simulink model "A4T2"  (R2017a)
settings: Solver=VariableStepAuto  StartTime=0.0  StopTime=w_base  MaxStep=1e-4*w_base  RelTol=1e-3
values from neighbouring files (symbols this model uses):
  alpha_l = 4    [parameters.m]
  epsilon = (Lsigma+LM)/Lsigma    (= 6.36273701566)    [parameters.m]
  I_base = 1    [parameters.m]
  K = sqrt(3/2)    [parameters.m]
  ki = alpha_c*(R+Ra)    (= 11.8344493889)    [parameters.m]
  ki_speed = alpha_speed*alpha_speed*J    (= 0.9756347394)    [parameters.m]
  kp = alpha_c*Lsigma    (= 1.69441359229)    [parameters.m]
  kp_speed = alpha_speed*J    (= 6.98439238374)    [parameters.m]
  lambda = 1.5    [parameters.m]
  lambda_delta = 0.2*1    (= 0.2)    [parameters.m]
  Lsigma = 0.2426    [parameters.m]
  Ra = alpha_c*Lsigma-R    (= 1.58785359229)    [parameters.m]
  Ra_speed = alpha_speed*J-b    (= 6.48439238374)    [parameters.m]
  RR = 0.06151    [parameters.m]
  Rs = 0.04505    [parameters.m]
  V_base = 1    [parameters.m]
  w_base = 314.59    [parameters.m]
libraries: simulink x1
settings Model: Creator=Oskar  LastModifiedBy=Callum

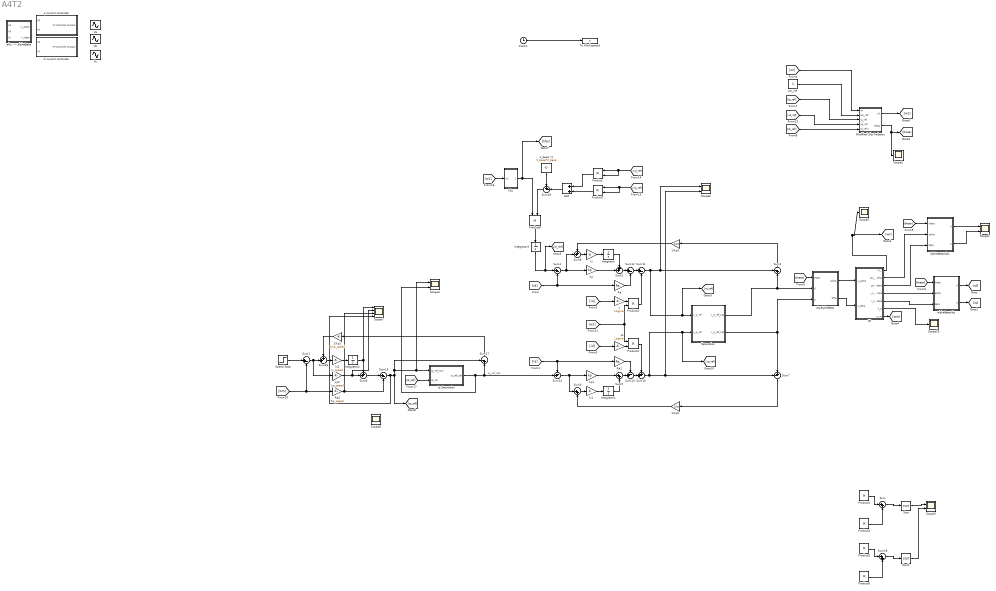
== system A4T2 ==
  note: iq_ref_sat
  1/kp1 : Gain  Gain=1/kp_speed
  1/kp2 : Gain  Gain=1/kp
  1/kp3 : Gain  Gain=1/kp
  Add : Sum
  Clock1 : Clock
  IM : Subsystem  mask{RR=0.06151, RS=0.04505, LM=1.301, Ls=0.2426, J=50, p=2, b_w1=0.5, b_w2=0}
      mask prompts: RR "Rr [p.u]"; RS "Rs [p.u]"; LM "Lm [p.u]"; Ls "Ls [p.u]"; J "J [p.u]"
  Integrator : Integrator
  Integrator1 : Integrator
  Integrator2 : Integrator
  Integrator3 : Integrator  InitialCondition=0.76863950807071483474250576479631  LimitOutput=on  UpperSaturationLimit=0.76863950807071483474250576479631  LowerSaturationLimit=0.1*I_base
  L : Gain  Gain=Lsigma
  L1 : Gain  Gain=Lsigma
  Modified Slip Relation : Subsystem
  Product{,1..8} (9 alike) : Product
  Ra : Gain  Gain=Ra
  Ra1 : Gain  Gain=Ra
  Ra2 : Gain  Gain=Ra_speed
  Saturation : Subsystem
  Scope{1,3..4,6,8} (5 alike) : Scope  NumInputPorts=2
  Scope10 : Scope
  Scope2 : Scope
  Scope5 : Scope
  Scope7 : Scope  NumInputPorts=4
  Speed Step : Step  Time=150  After=0.65  SampleTime=0
  Sqrt : Sqrt  SaturateOnIntegerOverflow=on
  Sqrt1 : Sqrt  SaturateOnIntegerOverflow=on
  Sum{,5,9,18} (4 alike) : Sum  Inputs=|++
  Sum{1,4,11..12,15} (5 alike) : Sum  Inputs=|+-
  Sum{3,6,8,10,16} (5 alike) : Sum  Inputs=++|
  Sum{2,7,13..14,17} (5 alike) : Sum  Inputs=-+|
  Sum19 : Sum  Inputs=+-|
  To Workspace1 : ToWorkspace  VariableName=t
      settings: MaxDataPoints=100000
  V_base^2 : Constant  Value=V_base*V_base
  Va : Sin  SampleTime=0
  Vb : Sin  Phase=2*pi/3  SampleTime=0
  Vc : Sin  Phase=4*pi/3  SampleTime=0
  abc --> alphaBeta : Subsystem
  alphaBeta/dq : Subsystem
  alphaBeta/dq1 : Subsystem
  d current controller : Subsystem
  dq/alphaBeta : Subsystem
  iq Saturation : Subsystem
  kfw : Subsystem
  ki : Gain  Gain=ki
  ki1 : Gain  Gain=ki
  ki2 : Gain  Gain=ki_speed
  kp : Gain  Gain=kp
  kp1 : Gain  Gain=kp
  kp2 : Gain  Gain=kp_speed
  psi_ref : Constant
  q current controller : Subsystem
  wires:
  Clock1/1 -> To Workspace1/1
  dq/alphaBeta/1(alpha) -> IM/1(u_alpha)
  dq/alphaBeta/2(beta) -> IM/2(u_beta)
  IM/4(i_s_s_alpha) -> alphaBeta/dq/2(alpha)
  IM/5(i_s_s_beta) -> alphaBeta/dq/3("beta ")
  alphaBeta/dq/1(d) -> [id]
  ki/1 -> Integrator/1
  Sum4/1 -> kp/1, Sum8/2
  [id] -> Ra/1, Sum4/2
  Sum14/1 -> kp1/1, Sum9/1
  ki1/1 -> Integrator1/1
  kp1/1 -> Sum5/1
  Integrator1/1 -> Sum5/2
  Sum7/1 -> 1/kp2/1
  Sum2/1 -> 1/kp3/1
  kp/1 -> Sum3/2
  Integrator/1 -> Sum3/1
  Sum8/1 -> ki/1
  1/kp3/1 -> Sum8/1
  Sum9/1 -> ki1/1
  1/kp2/1 -> Sum9/2
  [iq] -> L/1
  [id] -> L1/1
  Sum3/1 -> Sum12/1
  Sum12/1 -> Sum11/1
  Ra/1 -> Sum12/2
  Sum5/1 -> Sum13/2
  Sum13/1 -> Sum10/2
  Ra1/1 -> Sum13/1
  [iq] -> Ra1/1, Sum14/1
  IM/1(w_r) -> Scope5/1, [wr]
  Modified Slip Relation/2(theta) -> Scope2/1, [theta]
  [theta] -> dq/alphaBeta/1(theta)
  [theta] -> alphaBeta/dq/1(theta)
  Sum15/1 -> Scope7/4, Scope4/1, iq Saturation/1(iq_ref_nom), Sum17/1, [iq_ref]
  L/1 -> Product3/1
  Product3/1 -> Sum11/2
  [w1] -> Product3/2, Product4/1
  L1/1 -> Product4/2
  Product4/1 -> Sum10/1
  Saturation/1(v_d_ref_sat) -> Sum2/2, dq/alphaBeta/2(d)
  Saturation/2(v_q_ref_sat) -> dq/alphaBeta/3("q "), Sum7/2
  IM/2(psi_r_alpha) -> alphaBeta/dq1/2(alpha)
  IM/3(psi_r_beta) -> alphaBeta/dq1/3("beta ")
  [theta] -> alphaBeta/dq1/1(theta)
  Modified Slip Relation/1(w1) -> [w1]
  Speed Step/1 -> Sum1/1
  IM/7(w_m) -> [wm]
  [wm] -> Sum1/2, Ra2/1
  ki2/1 -> Integrator2/1
  Sum16/1 -> ki2/1
  kp2/1 -> Scope7/2, Sum6/2
  Integrator2/1 -> Sum6/1, Scope7/1
  Sum1/1 -> kp2/1, Sum16/2
  Sum6/1 -> Sum15/1
  Ra2/1 -> Sum15/2, Scope7/3
  1/kp1/1 -> Sum16/1
  Sum17/1 -> 1/kp1/1
  IM/6(T_e) -> Scope10/1
  Sum/1 -> Sqrt/1
  Product1/1 -> Sum/1
  Product2/1 -> Sum/2
  Sqrt/1 -> Scope3/1
  Sum18/1 -> Sqrt1/1
  Product6/1 -> Sum18/2
  Product5/1 -> Sum18/1
  Sqrt1/1 -> Scope3/2
  alphaBeta/dq/2(q) -> [iq]
  alphaBeta/dq1/1(d) -> Scope1/1
  alphaBeta/dq1/2(q) -> Scope1/2
  [id_ref] -> Modified Slip Relation/5(id_ref 1)
  [iq_ref] -> Modified Slip Relation/3("iq_ref ")
  [wr] -> Modified Slip Relation/1(wr)
  [vd_ref] -> Modified Slip Relation/4(vd_ref)
  V_base^2/1 -> Sum19/1
  Add/1 -> Sum19/2
  Product7/1 -> Add/2
  Product/1 -> Add/1
  [vq_ref] -> Product7/2, Product7/1
  [vd_ref] -> Product/2, Product/1
  [w1] -> kfw/1(w1)
  Product8/1 -> Integrator3/1
  Sum19/1 -> Product8/2
  iq Saturation/1(iq_ref_sat) -> Scope4/2, Sum17/2, Sum14/2
  [id_ref] -> iq Saturation/2(id_ref)
  psi_ref/1 -> Modified Slip Relation/2(psi_ref)
  kfw/1(kfw) -> Product8/1, [kfw]
  Sum11/1 -> [vd_ref], Saturation/1(v_d_ref), Scope6/1, Sum2/1
  Sum10/1 -> Saturation/2(v_q_ref), [vq_ref], Scope6/2, Sum7/1
  Integrator3/1 -> [id_ref], Sum4/1

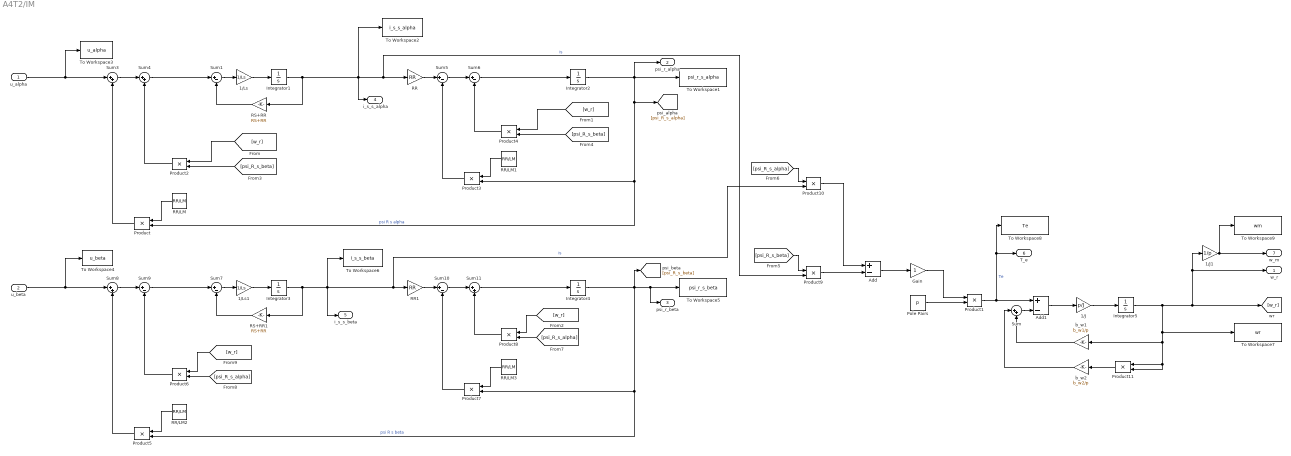
== system A4T2/IM ==
  u_alpha : Inport
  u_beta : Inport  Port=2
  1/J : Gain  Gain=p/J
  1/J1 : Gain  Gain=1/p
  1/Ls : Gain  Gain=1/Ls
  1/Ls1 : Gain  Gain=1/Ls
  Add : Sum  Inputs=+-
  Add1 : Sum  Inputs=+-
  Gain : Gain
  Integrator{1..5} (5 alike) : Integrator
  Pole Pairs : Constant  Value=p
  Product{,1..11} (12 alike) : Product  SaturateOnIntegerOverflow=on  InputSameDT=on  OutDataTypeStr=Inherit: Same as first input
  RR : Gain  Gain=RR
  RR/LM{,1..3} (4 alike) : Constant  Value=RR/LM
  RR1 : Gain  Gain=RR
  RS+RR : Gain  Gain=RS+RR
  RS+RR1 : Gain  Gain=RS+RR
  Sum{,3..4,8,11} (5 alike) : Sum  Inputs=|++
  Sum{1,5..7,9..10} (6 alike) : Sum  Inputs=|+-
  To Workspace1 : ToWorkspace  VariableName=psi_r_s_alpha
      settings: MaxDataPoints=100000
  To Workspace2 : ToWorkspace  VariableName=i_s_s_alpha
      settings: MaxDataPoints=100000
  To Workspace3 : ToWorkspace  VariableName=u_alpha
      settings: MaxDataPoints=100000
  To Workspace4 : ToWorkspace  VariableName=u_beta
      settings: MaxDataPoints=100000
  To Workspace5 : ToWorkspace  VariableName=psi_r_s_beta
      settings: MaxDataPoints=100000
  To Workspace6 : ToWorkspace  VariableName=i_s_s_beta
      settings: MaxDataPoints=100000
  To Workspace7 : ToWorkspace  VariableName=wr
      settings: MaxDataPoints=100000
  To Workspace8 : ToWorkspace  VariableName=Te
      settings: MaxDataPoints=100000
  To Workspace9 : ToWorkspace  VariableName=wm
      settings: MaxDataPoints=100000
  b_w1 : Gain  Gain=b_w1/p
  b_w2 : Gain  Gain=b_w2/p
  w_r : Outport
  psi_r_alpha : Outport  Port=2
  psi_r_beta : Outport  Port=3
  i_s_s_alpha : Outport  Port=4
  i_s_s_beta : Outport  Port=5
  T_e : Outport  Port=6
  w_m : Outport  Port=7
  wires:
  RR/LM1/1 -> Product3/1
  Product3/1 -> Sum5/2
  [psi_R_s_alpha] -> Product8/2
  1/Ls/1 -> Integrator1/1
  1/J/1 -> Integrator5/1
  Pole Pairs/1 -> Product1/2
  Add1/1 -> 1/J/1
  Sum1/1 -> 1/Ls/1
  Sum3/1 -> Sum4/1
  Sum4/1 -> Sum1/1
  Integrator2/1 -> psi_r_alpha/1, [psi_R_s_alpha], Product/2, Product3/2, To Workspace1/1  "psi R s alpha"
  RR/LM/1 -> Product/1
  Product10/1 -> Add/1
  Product9/1 -> Add/2
  Sum5/1 -> Sum6/1
  [psi_R_s_beta] -> Product2/2
  [w_r] -> Product2/1
  [w_r] -> Product6/1
  Product/1 -> Sum3/2
  Product1/1 -> To Workspace8/1, T_e/1, Add1/1  "Te"
  [w_r] -> Product8/1
  Sum6/1 -> Integrator2/1
  Add/1 -> Gain/1
  Product5/1 -> Sum8/2
  Sum11/1 -> Integrator4/1
  Integrator3/1 -> i_s_s_beta/1, Product10/2, RR1/1, To Workspace6/1, RS+RR1/1  "is"
  RR/LM3/1 -> Product7/1
  Sum9/1 -> Sum7/1
  RS+RR1/1 -> Sum7/2
  1/Ls1/1 -> Integrator3/1
  Sum8/1 -> Sum9/1
  Integrator4/1 -> [psi_R_s_beta], Product5/2, Product7/2, psi_r_beta/1, To Workspace5/1  "psi R s beta"
  RR1/1 -> Sum10/1
  Product8/1 -> Sum11/2
  u_beta/1 -> To Workspace4/1, Sum8/1
  Product6/1 -> Sum9/2
  Product7/1 -> Sum10/2
  Sum10/1 -> Sum11/1
  RR/LM2/1 -> Product5/1
  Sum7/1 -> 1/Ls1/1
  [psi_R_s_beta] -> Product9/1
  Integrator1/1 -> i_s_s_alpha/1, Product9/2, RR/1, To Workspace2/1, RS+RR/1  "is"
  Product4/1 -> Sum6/2
  u_alpha/1 -> Sum3/1, To Workspace3/1
  Gain/1 -> Product1/1
  [w_r] -> Product4/1
  [psi_R_s_alpha] -> Product10/1
  [psi_R_s_alpha] -> Product6/2
  [psi_R_s_beta] -> Product4/2
  RR/1 -> Sum5/1
  RS+RR/1 -> Sum1/2
  Product2/1 -> Sum4/2
  Sum/1 -> Add1/2
  b_w1/1 -> Sum/2
  b_w2/1 -> Sum/1
  Product11/1 -> b_w2/1
  Integrator5/1 -> 1/J1/1, w_r/1, [w_r], Product11/2, Product11/1, b_w1/1, To Workspace7/1
  1/J1/1 -> To Workspace9/1, w_m/1

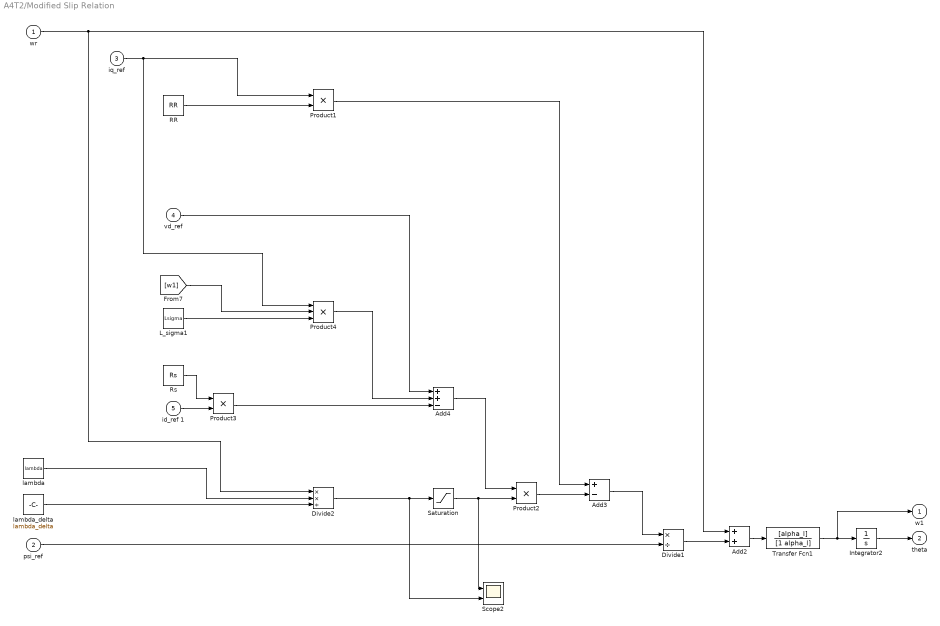
== system A4T2/Modified Slip Relation ==
  wr : Inport
  psi_ref : Inport  Port=2
  "iq_ref " : Inport  Port=3
  vd_ref : Inport  Port=4
  id_ref 1 : Inport  Port=5
  Add2 : Sum
  Add3 : Sum  Inputs=+-
  Add4 : Sum  Inputs=++-
  Divide1 : Product  Inputs=*/
  Divide2 : Product  Inputs=**/
  Integrator2 : Integrator
  L_sigma1 : Constant  Value=Lsigma
  Product1 : Product
  Product2 : Product
  Product3 : Product
  Product4 : Product  Inputs=3
  RR : Constant  Value=RR
  Rs : Constant  Value=Rs
  Saturation : Saturate  UpperLimit=lambda  LowerLimit=-lambda
  Scope2 : Scope  NumInputPorts=2
  Transfer Fcn1 : TransferFcn  Numerator=[alpha_l]  Denominator=[1 alpha_l]
  lambda : Constant  Value=lambda
  lambda_delta : Constant  Value=lambda_delta
  w1 : Outport
  theta : Outport  Port=2
  wires:
  Integrator2/1 -> theta/1
  Transfer Fcn1/1 -> w1/1, Integrator2/1
  Add2/1 -> Transfer Fcn1/1
  wr/1 -> Divide2/1, Add2/1
  Divide1/1 -> Add2/2
  Add3/1 -> Divide1/1
  psi_ref/1 -> Divide1/2
  "iq_ref "/1 -> Product4/1, Product1/1
  RR/1 -> Product1/2
  Product1/1 -> Add3/1
  Product2/1 -> Add3/2
  vd_ref/1 -> Add4/1
  Rs/1 -> Product3/1
  id_ref 1/1 -> Product3/2
  Product3/1 -> Add4/3
  L_sigma1/1 -> Product4/3
  [w1] -> Product4/2
  Product4/1 -> Add4/2
  Add4/1 -> Product2/1
  lambda/1 -> Divide2/2
  lambda_delta/1 -> Divide2/3
  Saturation/1 -> Scope2/1, Product2/2
  Divide2/1 -> Scope2/2, Saturation/1

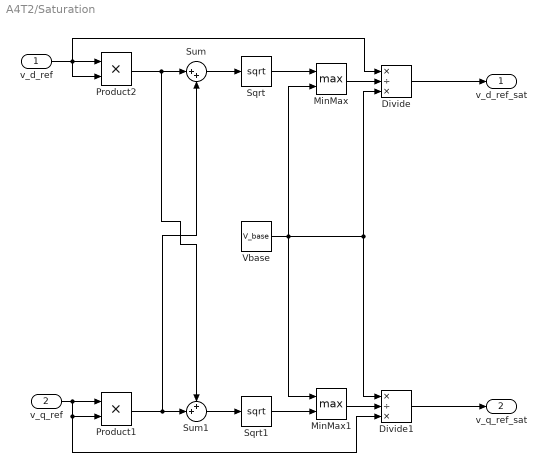
== system A4T2/Saturation ==
  v_d_ref : Inport
  v_q_ref : Inport  Port=2
  Divide : Product  Inputs=*/*
  Divide1 : Product  Inputs=*/*
  MinMax : MinMax  Function=max  Inputs=2
  MinMax1 : MinMax  Function=max  Inputs=2
  Product1 : Product
  Product2 : Product
  Sqrt : Sqrt  SaturateOnIntegerOverflow=on
  Sqrt1 : Sqrt  SaturateOnIntegerOverflow=on
  Sum : Sum  Inputs=|++
  Sum1 : Sum  Inputs=++|
  Vbase : Constant  Value=V_base
  v_d_ref_sat : Outport
  v_q_ref_sat : Outport  Port=2
  wires:
  Sum1/1 -> Sqrt1/1
  MinMax1/1 -> Divide1/2
  Sum/1 -> Sqrt/1
  Product2/1 -> Sum/1, Sum1/1
  MinMax/1 -> Divide/2
  Sqrt1/1 -> MinMax1/2
  Vbase/1 -> MinMax/2, Divide/3, Divide1/1, MinMax1/1
  Divide/1 -> v_d_ref_sat/1
  Divide1/1 -> v_q_ref_sat/1
  Product1/1 -> Sum/2, Sum1/2
  Sqrt/1 -> MinMax/1
  v_d_ref/1 -> Divide/1, Product2/2, Product2/1
  v_q_ref/1 -> Divide1/3, Product1/2, Product1/1

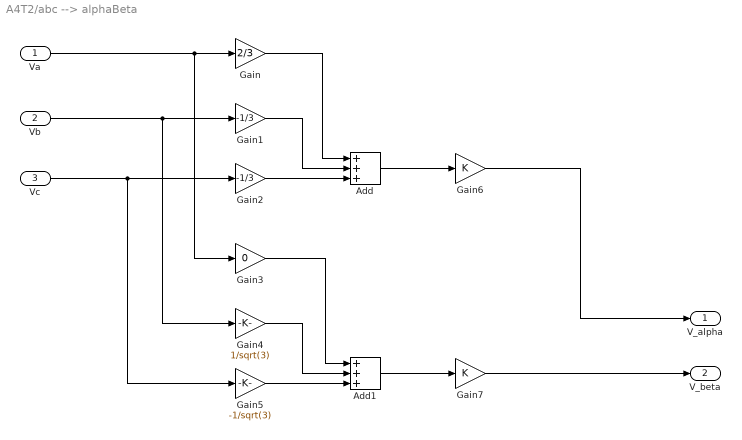
== system A4T2/abc --> alphaBeta ==
  Va : Inport
  Vb : Inport  Port=2
  Vc : Inport  Port=3
  Add : Sum  Inputs=+++
  Add1 : Sum  Inputs=+++
  Gain : Gain  Gain=2/3
  Gain1 : Gain  Gain=-1/3
  Gain2 : Gain  Gain=-1/3
  Gain3 : Gain  Gain=0
  Gain4 : Gain  Gain=1/sqrt(3)
  Gain5 : Gain  Gain=-1/sqrt(3)
  Gain6 : Gain  Gain=K
  Gain7 : Gain  Gain=K
  V_alpha : Outport
  V_beta : Outport  Port=2
  wires:
  Add/1 -> Gain6/1
  Va/1 -> Gain3/1, Gain/1
  Vc/1 -> Gain5/1, Gain2/1
  Vb/1 -> Gain4/1, Gain1/1
  Gain3/1 -> Add1/1
  Gain6/1 -> V_alpha/1
  Gain7/1 -> V_beta/1
  Add1/1 -> Gain7/1
  Gain1/1 -> Add/2
  Gain/1 -> Add/1
  Gain5/1 -> Add1/3
  Gain2/1 -> Add/3
  Gain4/1 -> Add1/2

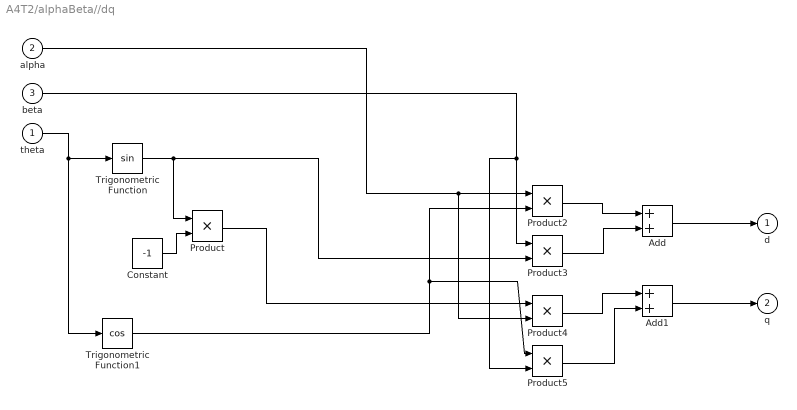
== system A4T2/alphaBeta//dq ==
  theta : Inport
  alpha : Inport  Port=2
  "beta " : Inport  Port=3
  Add : Sum
  Add1 : Sum
  Constant : Constant  Value=-1
  Product{,2..5} (5 alike) : Product
  Trigonometric Function : Trigonometry
  Trigonometric Function1 : Trigonometry  Operator=cos
  d : Outport
  q : Outport  Port=2
  wires:
  theta/1 -> Trigonometric Function1/1, Trigonometric Function/1
  Product4/1 -> Add1/1
  Product5/1 -> Add1/2
  Trigonometric Function1/1 -> Product2/2, Product5/1
  Product/1 -> Product4/1
  Trigonometric Function/1 -> Product/1, Product3/2
  Add1/1 -> q/1
  alpha/1 -> Product2/1, Product4/2
  "beta "/1 -> Product5/2, Product3/1
  Add/1 -> d/1
  Constant/1 -> Product/2
  Product2/1 -> Add/1
  Product3/1 -> Add/2

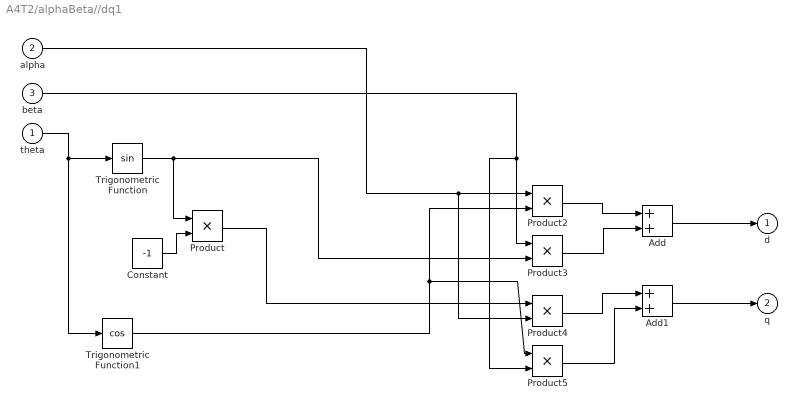
== system A4T2/alphaBeta//dq1 ==
  theta : Inport
  alpha : Inport  Port=2
  "beta " : Inport  Port=3
  Add : Sum
  Add1 : Sum
  Constant : Constant  Value=-1
  Product{,2..5} (5 alike) : Product
  Trigonometric Function : Trigonometry
  Trigonometric Function1 : Trigonometry  Operator=cos
  d : Outport
  q : Outport  Port=2
  wires:
  theta/1 -> Trigonometric Function1/1, Trigonometric Function/1
  Product4/1 -> Add1/1
  Product5/1 -> Add1/2
  Trigonometric Function1/1 -> Product2/2, Product5/1
  Product/1 -> Product4/1
  Trigonometric Function/1 -> Product/1, Product3/2
  Add1/1 -> q/1
  alpha/1 -> Product2/1, Product4/2
  "beta "/1 -> Product5/2, Product3/1
  Add/1 -> d/1
  Constant/1 -> Product/2
  Product2/1 -> Add/1
  Product3/1 -> Add/2

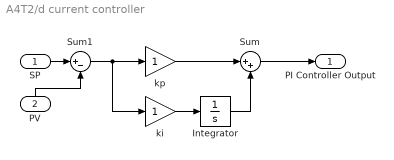
== system A4T2/d current controller ==
  SP : Inport
  PV : Inport  Port=2
  Integrator : Integrator
  Sum : Sum  Inputs=|++
  Sum1 : Sum  Inputs=|+-
  ki : Gain
  kp : Gain
  PI Controller Output : Outport
  wires:
  ki/1 -> Integrator/1
  kp/1 -> Sum/1
  Integrator/1 -> Sum/2
  Sum/1 -> PI Controller Output/1
  Sum1/1 -> ki/1, kp/1
  PV/1 -> Sum1/2
  SP/1 -> Sum1/1

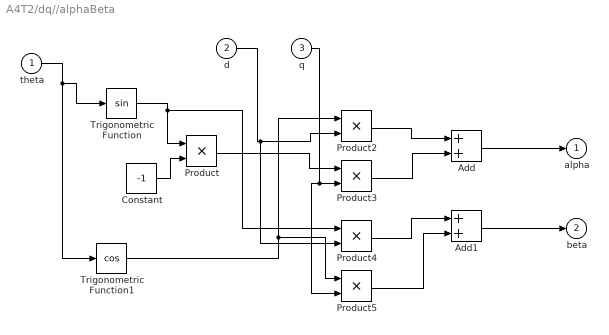
== system A4T2/dq//alphaBeta ==
  theta : Inport
  d : Inport  Port=2
  "q " : Inport  Port=3
  Add : Sum
  Add1 : Sum
  Constant : Constant  Value=-1
  Product{,2..5} (5 alike) : Product
  Trigonometric Function : Trigonometry
  Trigonometric Function1 : Trigonometry  Operator=cos
  alpha : Outport
  beta : Outport  Port=2
  wires:
  theta/1 -> Trigonometric Function1/1, Trigonometric Function/1
  Product4/1 -> Add1/1
  Product5/1 -> Add1/2
  Trigonometric Function/1 -> Product4/1, Product/1
  Add1/1 -> beta/1
  Add/1 -> alpha/1
  Constant/1 -> Product/2
  Product2/1 -> Add/1
  Product3/1 -> Add/2
  Trigonometric Function1/1 -> Product5/1, Product2/1
  Product/1 -> Product3/1
  d/1 -> Product4/2, Product2/2
  "q "/1 -> Product3/2, Product5/2

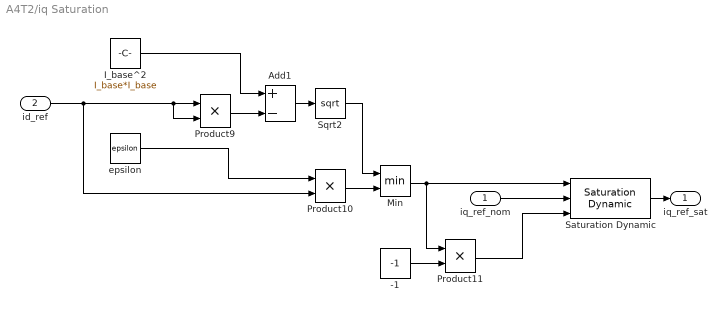
== system A4T2/iq Saturation ==
  iq_ref_nom : Inport
  id_ref : Inport  Port=2
  "-1 " : Constant  Value=-1
  Add1 : Sum  Inputs=+-
  I_base^2 : Constant  Value=I_base*I_base
  Min : MinMax  Inputs=2
  Product10 : Product
  Product11 : Product
  Product9 : Product
  Saturation Dynamic : simulink/Discontinuities/Saturation Dynamic  OutMin=[]  OutMax=[]  OutDataTypeStr=Inherit: Same as second input  OutDataType=fixdt(1, 16)  OutScaling=2^-10  DoSatur=off
  Sqrt2 : Sqrt  SaturateOnIntegerOverflow=on
  epsilon : Constant  Value=epsilon
  iq_ref_sat : Outport
  wires:
  Min/1 -> Product11/1, Saturation Dynamic/1
  Product11/1 -> Saturation Dynamic/3
  "-1 "/1 -> Product11/2
  id_ref/1 -> Product10/2, Product9/1, Product9/2
  epsilon/1 -> Product10/1
  I_base^2/1 -> Add1/1
  Product9/1 -> Add1/2
  Sqrt2/1 -> Min/1
  iq_ref_nom/1 -> Saturation Dynamic/2
  Saturation Dynamic/1 -> iq_ref_sat/1
  Product10/1 -> Min/2
  Add1/1 -> Sqrt2/1

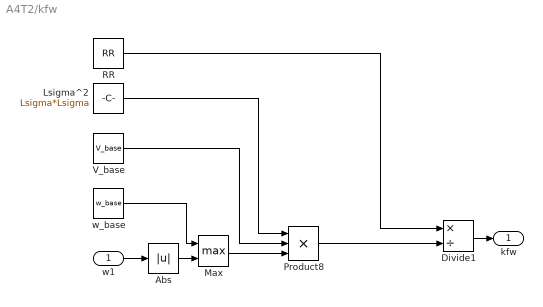
== system A4T2/kfw ==
  w1 : Inport
  Abs : Abs
  Divide1 : Product  Inputs=*/
  Lsigma^2 : Constant  Value=Lsigma*Lsigma
  Max : MinMax  Function=max  Inputs=2
  Product8 : Product  Inputs=3
  RR : Constant  Value=RR
  V_base : Constant  Value=V_base
  w_base : Constant  Value=w_base
  kfw : Outport
  wires:
  w_base/1 -> Max/1
  V_base/1 -> Product8/2
  Max/1 -> Product8/3
  Lsigma^2/1 -> Product8/1
  RR/1 -> Divide1/1
  Divide1/1 -> kfw/1
  Product8/1 -> Divide1/2
  w1/1 -> Abs/1
  Abs/1 -> Max/2

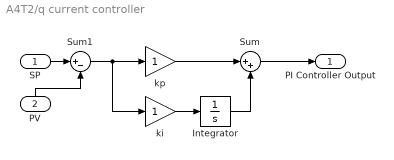
== system A4T2/q current controller ==
  SP : Inport
  PV : Inport  Port=2
  Integrator : Integrator
  Sum : Sum  Inputs=|++
  Sum1 : Sum  Inputs=|+-
  ki : Gain
  kp : Gain
  PI Controller Output : Outport
  wires:
  ki/1 -> Integrator/1
  kp/1 -> Sum/1
  Integrator/1 -> Sum/2
  Sum/1 -> PI Controller Output/1
  Sum1/1 -> ki/1, kp/1
  PV/1 -> Sum1/2
  SP/1 -> Sum1/1
